simulink library "MEKF_Inputs_lib"  (R2018b)
settings: Solver=VariableStepAuto  StartTime=0.0  StopTime=10.0  RelTol=1e-3
libraries: dspindex x4, sunsensor2body_lib x1
settings Model: Creator=kylle  LastModifiedBy=kashton6

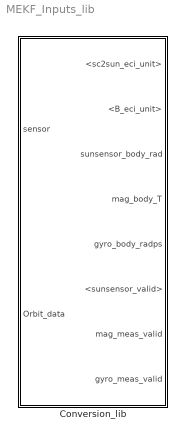
== system MEKF_Inputs_lib ==
  Conversion_lib : Subsystem

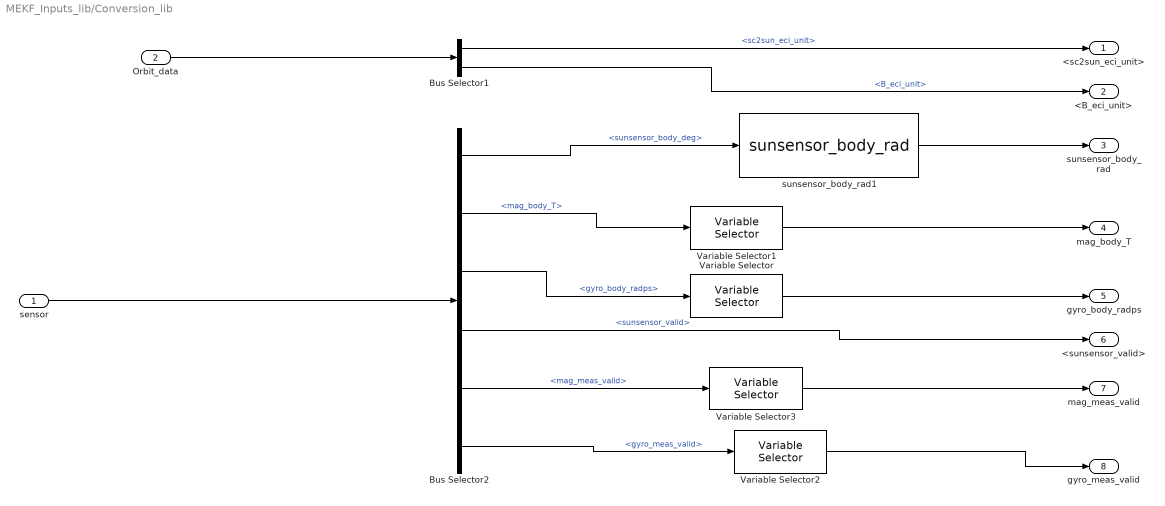
== system MEKF_Inputs_lib/Conversion_lib ==
  sensor : Inport
  Orbit_data : Inport  Port=2
  Bus Selector1 : BusSelector  OutputSignals=sc2sun_eci_unit,B_eci_unit
  Bus Selector2 : BusSelector  OutputSignals=sunsensor_body_deg,mag_body_T,gyro_body_radps,sunsensor_valid,mag_meas_valid,gyro_meas_valid
  Variable Selector : dspindex/Variable Selector  NumInputs=1  rowsOrCols=Columns  IdxMode=Fixed  Elements=[1]  ZerOneIdxMode=One-based  errmode=Clip Index  FillMode=off  FillValues=0
  Variable Selector1 : dspindex/Variable Selector  NumInputs=1  rowsOrCols=Columns  IdxMode=Fixed  Elements=[1]  ZerOneIdxMode=One-based  errmode=Clip Index  FillMode=off  FillValues=0
  Variable Selector2 : dspindex/Variable Selector  NumInputs=1  rowsOrCols=Rows  IdxMode=Fixed  Elements=[1]  ZerOneIdxMode=One-based  errmode=Clip Index  FillMode=off  FillValues=0
  Variable Selector3 : dspindex/Variable Selector  NumInputs=1  rowsOrCols=Rows  IdxMode=Fixed  Elements=[1]  ZerOneIdxMode=One-based  errmode=Clip Index  FillMode=off  FillValues=0
  sunsensor_body_rad1 : sunsensor2body_lib/sunsensor_body_rad  SystemSampleTime=-1
  <sc2sun_eci_unit> : Outport
  <B_eci_unit> : Outport  Port=2
  sunsensor_body_rad : Outport  Port=3
  mag_body_T : Outport  Port=4
  gyro_body_radps : Outport  Port=5
  <sunsensor_valid> : Outport  Port=6
  mag_meas_valid : Outport  Port=7
  gyro_meas_valid : Outport  Port=8
  wires:
  Bus Selector2/3 -> Variable Selector/1  "<gyro_body_radps>"
  Bus Selector1/2 -> <B_eci_unit>/1  "<B_eci_unit>"
  Bus Selector2/1 -> sunsensor_body_rad1/1  "<sunsensor_body_deg>"
  Bus Selector2/2 -> Variable Selector1/1  "<mag_body_T>"
  sunsensor_body_rad1/1 -> sunsensor_body_rad/1
  Bus Selector2/5 -> Variable Selector3/1  "<mag_meas_valid>"
  Bus Selector2/6 -> Variable Selector2/1  "<gyro_meas_valid>"
  sensor/1 -> Bus Selector2/1
  Variable Selector1/1 -> mag_body_T/1
  Variable Selector2/1 -> gyro_meas_valid/1
  Bus Selector1/1 -> <sc2sun_eci_unit>/1  "<sc2sun_eci_unit>"
  Bus Selector2/4 -> <sunsensor_valid>/1  "<sunsensor_valid>"
  Orbit_data/1 -> Bus Selector1/1
  Variable Selector/1 -> gyro_body_radps/1
  Variable Selector3/1 -> mag_meas_valid/1
